simulink model "CarSim_SCANeR_UDP_LKA_THESIS"  (R2019a)
settings: Solver=FixedStepDiscrete  StartTime=0.0  StopTime=inf  FixedStep=0.001  RelTol=1e-3  EnableMultiTasking=on
undefined symbols (not defined in the file or in its folder): DiscIntNeverNeededParam
libraries: simulink x11, xpcutilitieslib x2, xpcrtudplib x2, dspnetwork x1
(part 2 of 2)

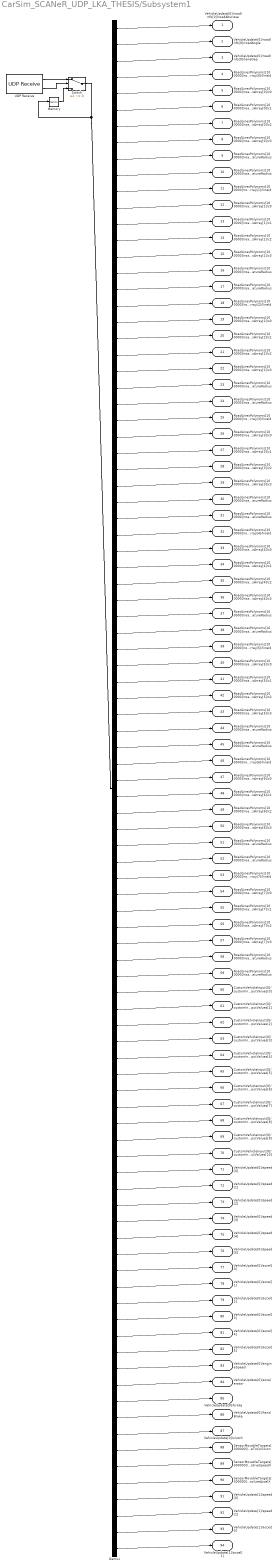
== system CarSim_SCANeR_UDP_LKA_THESIS/Subsystem1 ==
  Demux : Demux  Outputs=94
  Memory : Memory  InheritSampleTime=on
  Switch : Switch  Criteria=u2 ~= 0
  UDP Receive : dspnetwork/UDP Receive  localURL='0.0.0.0'  localPort=8193  remoteURL='0.0.0.0'  remotePort=-1  recvBufferSize=752  dims=94  signalDatatype=double  isComplex=off  isVarSize=off  showBlockingTime=on  blockingTime=0  sampletime=0.01  blockPlatform=HOST
      settings: SourceProductName=Simulink
  VehicleUpdate[0]/roadInfo[0]/roadAbscissa : Outport
  VehicleUpdate[0]/roadInfo[0]/roadAngle : Outport  Port=2
  VehicleUpdate[0]/roadInfo[0]/laneGap : Outport  Port=3
  RoadLinesPolynoms[100000]/roadLinesPolynomsArray[0]/lineId : Outport  Port=4
  RoadLinesPolynoms[100000]/roadLinesPolynomsArray[0]/c0 : Outport  Port=5
  RoadLinesPolynoms[100000]/roadLinesPolynomsArray[0]/c1 : Outport  Port=6
  RoadLinesPolynoms[100000]/roadLinesPolynomsArray[0]/c2 : Outport  Port=7
  RoadLinesPolynoms[100000]/roadLinesPolynomsArray[0]/c3 : Outport  Port=8
  RoadLinesPolynoms[100000]/roadLinesPolynomsArray[0]/curvatureRadius : Outport  Port=9
  RoadLinesPolynoms[100000]/roadLinesPolynomsArray[0]/estimatedCurvatureRadius : Outport  Port=10
  RoadLinesPolynoms[100000]/roadLinesPolynomsArray[1]/lineId : Outport  Port=11
  RoadLinesPolynoms[100000]/roadLinesPolynomsArray[1]/c0 : Outport  Port=12
  RoadLinesPolynoms[100000]/roadLinesPolynomsArray[1]/c1 : Outport  Port=13
  RoadLinesPolynoms[100000]/roadLinesPolynomsArray[1]/c2 : Outport  Port=14
  RoadLinesPolynoms[100000]/roadLinesPolynomsArray[1]/c3 : Outport  Port=15
  RoadLinesPolynoms[100000]/roadLinesPolynomsArray[1]/curvatureRadius : Outport  Port=16
  RoadLinesPolynoms[100000]/roadLinesPolynomsArray[1]/estimatedCurvatureRadius : Outport  Port=17
  RoadLinesPolynoms[100000]/roadLinesPolynomsArray[2]/lineId : Outport  Port=18
  RoadLinesPolynoms[100000]/roadLinesPolynomsArray[2]/c0 : Outport  Port=19
  RoadLinesPolynoms[100000]/roadLinesPolynomsArray[2]/c1 : Outport  Port=20
  RoadLinesPolynoms[100000]/roadLinesPolynomsArray[2]/c2 : Outport  Port=21
  RoadLinesPolynoms[100000]/roadLinesPolynomsArray[2]/c3 : Outport  Port=22
  RoadLinesPolynoms[100000]/roadLinesPolynomsArray[2]/curvatureRadius : Outport  Port=23
  RoadLinesPolynoms[100000]/roadLinesPolynomsArray[2]/estimatedCurvatureRadius : Outport  Port=24
  RoadLinesPolynoms[100000]/roadLinesPolynomsArray[3]/lineId : Outport  Port=25
  RoadLinesPolynoms[100000]/roadLinesPolynomsArray[3]/c0 : Outport  Port=26
  RoadLinesPolynoms[100000]/roadLinesPolynomsArray[3]/c1 : Outport  Port=27
  RoadLinesPolynoms[100000]/roadLinesPolynomsArray[3]/c2 : Outport  Port=28
  RoadLinesPolynoms[100000]/roadLinesPolynomsArray[3]/c3 : Outport  Port=29
  RoadLinesPolynoms[100000]/roadLinesPolynomsArray[3]/curvatureRadius : Outport  Port=30
  RoadLinesPolynoms[100000]/roadLinesPolynomsArray[3]/estimatedCurvatureRadius : Outport  Port=31
  RoadLinesPolynoms[100000]/roadLinesPolynomsArray[4]/lineId : Outport  Port=32
  RoadLinesPolynoms[100000]/roadLinesPolynomsArray[4]/c0 : Outport  Port=33
  RoadLinesPolynoms[100000]/roadLinesPolynomsArray[4]/c1 : Outport  Port=34
  RoadLinesPolynoms[100000]/roadLinesPolynomsArray[4]/c2 : Outport  Port=35
  RoadLinesPolynoms[100000]/roadLinesPolynomsArray[4]/c3 : Outport  Port=36
  RoadLinesPolynoms[100000]/roadLinesPolynomsArray[4]/curvatureRadius : Outport  Port=37
  RoadLinesPolynoms[100000]/roadLinesPolynomsArray[4]/estimatedCurvatureRadius : Outport  Port=38
  RoadLinesPolynoms[100000]/roadLinesPolynomsArray[5]/lineId : Outport  Port=39
  RoadLinesPolynoms[100000]/roadLinesPolynomsArray[5]/c0 : Outport  Port=40
  RoadLinesPolynoms[100000]/roadLinesPolynomsArray[5]/c1 : Outport  Port=41
  RoadLinesPolynoms[100000]/roadLinesPolynomsArray[5]/c2 : Outport  Port=42
  RoadLinesPolynoms[100000]/roadLinesPolynomsArray[5]/c3 : Outport  Port=43
  RoadLinesPolynoms[100000]/roadLinesPolynomsArray[5]/curvatureRadius : Outport  Port=44
  RoadLinesPolynoms[100000]/roadLinesPolynomsArray[5]/estimatedCurvatureRadius : Outport  Port=45
  RoadLinesPolynoms[100000]/roadLinesPolynomsArray[6]/lineId : Outport  Port=46
  RoadLinesPolynoms[100000]/roadLinesPolynomsArray[6]/c0 : Outport  Port=47
  RoadLinesPolynoms[100000]/roadLinesPolynomsArray[6]/c1 : Outport  Port=48
  RoadLinesPolynoms[100000]/roadLinesPolynomsArray[6]/c2 : Outport  Port=49
  RoadLinesPolynoms[100000]/roadLinesPolynomsArray[6]/c3 : Outport  Port=50
  RoadLinesPolynoms[100000]/roadLinesPolynomsArray[6]/curvatureRadius : Outport  Port=51
  RoadLinesPolynoms[100000]/roadLinesPolynomsArray[6]/estimatedCurvatureRadius : Outport  Port=52
  RoadLinesPolynoms[100000]/roadLinesPolynomsArray[7]/lineId : Outport  Port=53
  RoadLinesPolynoms[100000]/roadLinesPolynomsArray[7]/c0 : Outport  Port=54
  RoadLinesPolynoms[100000]/roadLinesPolynomsArray[7]/c1 : Outport  Port=55
  RoadLinesPolynoms[100000]/roadLinesPolynomsArray[7]/c2 : Outport  Port=56
  RoadLinesPolynoms[100000]/roadLinesPolynomsArray[7]/c3 : Outport  Port=57
  RoadLinesPolynoms[100000]/roadLinesPolynomsArray[7]/curvatureRadius : Outport  Port=58
  RoadLinesPolynoms[100000]/roadLinesPolynomsArray[7]/estimatedCurvatureRadius : Outport  Port=59
  CustomVehicleInput[0]/customInputValues[0] : Outport  Port=60
  CustomVehicleInput[0]/customInputValues[1] : Outport  Port=61
  CustomVehicleInput[0]/customInputValues[2] : Outport  Port=62
  CustomVehicleInput[0]/customInputValues[3] : Outport  Port=63
  CustomVehicleInput[0]/customInputValues[4] : Outport  Port=64
  CustomVehicleInput[0]/customInputValues[5] : Outport  Port=65
  CustomVehicleInput[0]/customInputValues[6] : Outport  Port=66
  CustomVehicleInput[0]/customInputValues[7] : Outport  Port=67
  CustomVehicleInput[0]/customInputValues[8] : Outport  Port=68
  CustomVehicleInput[0]/customInputValues[9] : Outport  Port=69
  CustomVehicleInput[0]/customInputValues[10] : Outport  Port=70
  VehicleUpdate[0]/speed[0] : Outport  Port=71
  VehicleUpdate[0]/speed[1] : Outport  Port=72
  VehicleUpdate[0]/speed[2] : Outport  Port=73
  VehicleUpdate[0]/speed[3] : Outport  Port=74
  VehicleUpdate[0]/speed[4] : Outport  Port=75
  VehicleUpdate[0]/speed[5] : Outport  Port=76
  VehicleUpdate[0]/accel[0] : Outport  Port=77
  VehicleUpdate[0]/accel[1] : Outport  Port=78
  VehicleUpdate[0]/accel[2] : Outport  Port=79
  VehicleUpdate[0]/accel[3] : Outport  Port=80
  VehicleUpdate[0]/accel[4] : Outport  Port=81
  VehicleUpdate[0]/accel[5] : Outport  Port=82
  VehicleUpdate[0]/engineSpeed : Outport  Port=83
  VehicleUpdate[0]/accelerator : Outport  Port=84
  VehicleUpdate[0]/brake : Outport  Port=85
  VehicleUpdate[0]/handBrake : Outport  Port=86
  VehicleUpdate[0]/clutch : Outport  Port=87
  SensorMovableTargets[300000]/targetsArray[0]/distanceToCollision : Outport  Port=88
  SensorMovableTargets[300000]/targetsArray[0]/relativeSpeedX : Outport  Port=89
  SensorMovableTargets[300000]/targetsArray[0]/absoluteAccelX : Outport  Port=90
  VehicleUpdate[1]/speed[0] : Outport  Port=91
  VehicleUpdate[1]/speed[1] : Outport  Port=92
  VehicleUpdate[1]/accel[0] : Outport  Port=93
  VehicleUpdate[1]/accel[1] : Outport  Port=94
  wires:
  UDP Receive/1 -> Switch/1
  Demux/1 -> VehicleUpdate[0]/roadInfo[0]/roadAbscissa/1
  Demux/2 -> VehicleUpdate[0]/roadInfo[0]/roadAngle/1
  Demux/3 -> VehicleUpdate[0]/roadInfo[0]/laneGap/1
  Demux/4 -> RoadLinesPolynoms[100000]/roadLinesPolynomsArray[0]/lineId/1
  Demux/5 -> RoadLinesPolynoms[100000]/roadLinesPolynomsArray[0]/c0/1
  Demux/6 -> RoadLinesPolynoms[100000]/roadLinesPolynomsArray[0]/c1/1
  Demux/7 -> RoadLinesPolynoms[100000]/roadLinesPolynomsArray[0]/c2/1
  Demux/8 -> RoadLinesPolynoms[100000]/roadLinesPolynomsArray[0]/c3/1
  Demux/9 -> RoadLinesPolynoms[100000]/roadLinesPolynomsArray[0]/curvatureRadius/1
  Demux/10 -> RoadLinesPolynoms[100000]/roadLinesPolynomsArray[0]/estimatedCurvatureRadius/1
  Demux/11 -> RoadLinesPolynoms[100000]/roadLinesPolynomsArray[1]/lineId/1
  Demux/12 -> RoadLinesPolynoms[100000]/roadLinesPolynomsArray[1]/c0/1
  Demux/13 -> RoadLinesPolynoms[100000]/roadLinesPolynomsArray[1]/c1/1
  Demux/14 -> RoadLinesPolynoms[100000]/roadLinesPolynomsArray[1]/c2/1
  Demux/15 -> RoadLinesPolynoms[100000]/roadLinesPolynomsArray[1]/c3/1
  Demux/16 -> RoadLinesPolynoms[100000]/roadLinesPolynomsArray[1]/curvatureRadius/1
  Demux/17 -> RoadLinesPolynoms[100000]/roadLinesPolynomsArray[1]/estimatedCurvatureRadius/1
  Demux/18 -> RoadLinesPolynoms[100000]/roadLinesPolynomsArray[2]/lineId/1
  Demux/19 -> RoadLinesPolynoms[100000]/roadLinesPolynomsArray[2]/c0/1
  Demux/20 -> RoadLinesPolynoms[100000]/roadLinesPolynomsArray[2]/c1/1
  Demux/21 -> RoadLinesPolynoms[100000]/roadLinesPolynomsArray[2]/c2/1
  Demux/22 -> RoadLinesPolynoms[100000]/roadLinesPolynomsArray[2]/c3/1
  Demux/23 -> RoadLinesPolynoms[100000]/roadLinesPolynomsArray[2]/curvatureRadius/1
  Demux/24 -> RoadLinesPolynoms[100000]/roadLinesPolynomsArray[2]/estimatedCurvatureRadius/1
  Demux/25 -> RoadLinesPolynoms[100000]/roadLinesPolynomsArray[3]/lineId/1
  Demux/26 -> RoadLinesPolynoms[100000]/roadLinesPolynomsArray[3]/c0/1
  Demux/27 -> RoadLinesPolynoms[100000]/roadLinesPolynomsArray[3]/c1/1
  Demux/28 -> RoadLinesPolynoms[100000]/roadLinesPolynomsArray[3]/c2/1
  Demux/29 -> RoadLinesPolynoms[100000]/roadLinesPolynomsArray[3]/c3/1
  Demux/30 -> RoadLinesPolynoms[100000]/roadLinesPolynomsArray[3]/curvatureRadius/1
  Demux/31 -> RoadLinesPolynoms[100000]/roadLinesPolynomsArray[3]/estimatedCurvatureRadius/1
  Demux/32 -> RoadLinesPolynoms[100000]/roadLinesPolynomsArray[4]/lineId/1
  Demux/33 -> RoadLinesPolynoms[100000]/roadLinesPolynomsArray[4]/c0/1
  Demux/34 -> RoadLinesPolynoms[100000]/roadLinesPolynomsArray[4]/c1/1
  Demux/35 -> RoadLinesPolynoms[100000]/roadLinesPolynomsArray[4]/c2/1
  Demux/36 -> RoadLinesPolynoms[100000]/roadLinesPolynomsArray[4]/c3/1
  Demux/37 -> RoadLinesPolynoms[100000]/roadLinesPolynomsArray[4]/curvatureRadius/1
  Demux/38 -> RoadLinesPolynoms[100000]/roadLinesPolynomsArray[4]/estimatedCurvatureRadius/1
  Demux/39 -> RoadLinesPolynoms[100000]/roadLinesPolynomsArray[5]/lineId/1
  Demux/40 -> RoadLinesPolynoms[100000]/roadLinesPolynomsArray[5]/c0/1
  Demux/41 -> RoadLinesPolynoms[100000]/roadLinesPolynomsArray[5]/c1/1
  Demux/42 -> RoadLinesPolynoms[100000]/roadLinesPolynomsArray[5]/c2/1
  Demux/43 -> RoadLinesPolynoms[100000]/roadLinesPolynomsArray[5]/c3/1
  Demux/44 -> RoadLinesPolynoms[100000]/roadLinesPolynomsArray[5]/curvatureRadius/1
  Demux/45 -> RoadLinesPolynoms[100000]/roadLinesPolynomsArray[5]/estimatedCurvatureRadius/1
  Demux/46 -> RoadLinesPolynoms[100000]/roadLinesPolynomsArray[6]/lineId/1
  Demux/47 -> RoadLinesPolynoms[100000]/roadLinesPolynomsArray[6]/c0/1
  Demux/48 -> RoadLinesPolynoms[100000]/roadLinesPolynomsArray[6]/c1/1
  Demux/49 -> RoadLinesPolynoms[100000]/roadLinesPolynomsArray[6]/c2/1
  Demux/50 -> RoadLinesPolynoms[100000]/roadLinesPolynomsArray[6]/c3/1
  Demux/51 -> RoadLinesPolynoms[100000]/roadLinesPolynomsArray[6]/curvatureRadius/1
  Demux/52 -> RoadLinesPolynoms[100000]/roadLinesPolynomsArray[6]/estimatedCurvatureRadius/1
  Demux/53 -> RoadLinesPolynoms[100000]/roadLinesPolynomsArray[7]/lineId/1
  Demux/54 -> RoadLinesPolynoms[100000]/roadLinesPolynomsArray[7]/c0/1
  Demux/55 -> RoadLinesPolynoms[100000]/roadLinesPolynomsArray[7]/c1/1
  Demux/56 -> RoadLinesPolynoms[100000]/roadLinesPolynomsArray[7]/c2/1
  Demux/57 -> RoadLinesPolynoms[100000]/roadLinesPolynomsArray[7]/c3/1
  Demux/58 -> RoadLinesPolynoms[100000]/roadLinesPolynomsArray[7]/curvatureRadius/1
  Demux/59 -> RoadLinesPolynoms[100000]/roadLinesPolynomsArray[7]/estimatedCurvatureRadius/1
  Demux/60 -> CustomVehicleInput[0]/customInputValues[0]/1
  Demux/61 -> CustomVehicleInput[0]/customInputValues[1]/1
  Demux/62 -> CustomVehicleInput[0]/customInputValues[2]/1
  Demux/63 -> CustomVehicleInput[0]/customInputValues[3]/1
  Demux/64 -> CustomVehicleInput[0]/customInputValues[4]/1
  Demux/65 -> CustomVehicleInput[0]/customInputValues[5]/1
  Demux/66 -> CustomVehicleInput[0]/customInputValues[6]/1
  Demux/67 -> CustomVehicleInput[0]/customInputValues[7]/1
  Demux/68 -> CustomVehicleInput[0]/customInputValues[8]/1
  Demux/69 -> CustomVehicleInput[0]/customInputValues[9]/1
  Demux/70 -> CustomVehicleInput[0]/customInputValues[10]/1
  Demux/71 -> VehicleUpdate[0]/speed[0]/1
  Demux/72 -> VehicleUpdate[0]/speed[1]/1
  Demux/73 -> VehicleUpdate[0]/speed[2]/1
  Demux/74 -> VehicleUpdate[0]/speed[3]/1
  Demux/75 -> VehicleUpdate[0]/speed[4]/1
  Demux/76 -> VehicleUpdate[0]/speed[5]/1
  Demux/77 -> VehicleUpdate[0]/accel[0]/1
  Demux/78 -> VehicleUpdate[0]/accel[1]/1
  Demux/79 -> VehicleUpdate[0]/accel[2]/1
  Demux/80 -> VehicleUpdate[0]/accel[3]/1
  Demux/81 -> VehicleUpdate[0]/accel[4]/1
  Demux/82 -> VehicleUpdate[0]/accel[5]/1
  Demux/83 -> VehicleUpdate[0]/engineSpeed/1
  Demux/84 -> VehicleUpdate[0]/accelerator/1
  Demux/85 -> VehicleUpdate[0]/brake/1
  Demux/86 -> VehicleUpdate[0]/handBrake/1
  Demux/87 -> VehicleUpdate[0]/clutch/1
  Demux/88 -> SensorMovableTargets[300000]/targetsArray[0]/distanceToCollision/1
  Demux/89 -> SensorMovableTargets[300000]/targetsArray[0]/relativeSpeedX/1
  Demux/90 -> SensorMovableTargets[300000]/targetsArray[0]/absoluteAccelX/1
  Demux/91 -> VehicleUpdate[1]/speed[0]/1
  Demux/92 -> VehicleUpdate[1]/speed[1]/1
  Demux/93 -> VehicleUpdate[1]/accel[0]/1
  Demux/94 -> VehicleUpdate[1]/accel[1]/1
  UDP Receive/2 -> Switch/2
  Switch/1 -> Memory/1, Demux/1
  Memory/1 -> Switch/3

== system CarSim_SCANeR_UDP_LKA_THESIS/LaneKeep/Subsystem ==
  In1 : Inport
  Enable : EnablePort
  S-Function : S-Function  FunctionName=casadi_fun_lka  Parameters='lka.casadi', 'lka'  SFunctionDeploymentMode=off  EnableBusSupport=off
  Steer : Outport
  wires:
  In1/1 -> S-Function/1
  S-Function/1 -> Steer/1  "Steer"

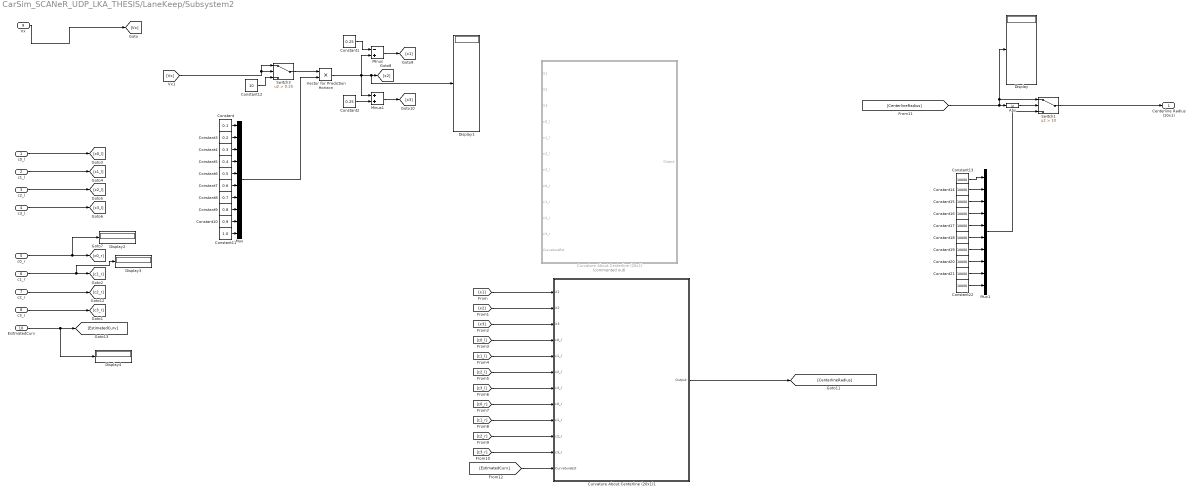
== system CarSim_SCANeR_UDP_LKA_THESIS/LaneKeep/Subsystem2 ==
  c0_l : Inport
  c1_l : Inport  Port=2
  c2_l : Inport  Port=3
  c3_l : Inport  Port=4
  c0_r : Inport  Port=5
  c1_r : Inport  Port=6
  c2_r : Inport  Port=7
  c3_r : Inport  Port=8
  Vx : Inport  Port=9
  EsitmatedCurv : Inport  Port=10
  Abs : Abs
  Constant : Constant  Value=0.1
  Constant1 : Constant  Value=0.25
  Constant10 : Constant  Value=0.9
  Constant11 : Constant  Value=1.0
  Constant12 : Constant  Value=10
  Constant{13..22} (10 alike) : Constant  Value=10000
  Constant2 : Constant  Value=0.25
  Constant3 : Constant  Value=0.2
  Constant4 : Constant  Value=0.3
  Constant5 : Constant  Value=0.4
  Constant6 : Constant  Value=0.5
  Constant7 : Constant  Value=0.6
  Constant8 : Constant  Value=0.7
  Constant9 : Constant  Value=0.8
  Curvature About Centerline (20x1) : Subsystem  Commented=on  TreatAsAtomicUnit=on
  Curvature About Centerline (20x1)1 : Subsystem
      mask help: Simulink:masks:GenSFuncDesc_MD
      mask Help: eval('feval(''rtwprivate'',''rtwhelpview'',''rtw_sfcn_block'')');
  Display{,1..4} (5 alike) : Display
  Minus : Sum  Inputs=-+
  Minus1 : Sum
  Mux : Mux  Inputs=10
  Mux1 : Mux  Inputs=10
  Switch1 : Switch  Criteria=u2 > Threshold  Threshold=10
  Switch3 : Switch  Criteria=u2 > Threshold  Threshold=0.25
  Vector for Prediction Horizon : Product  Inputs=**
  Centerline Radius (10x1) : Outport  VectorParamsAs1DForOutWhenUnconnected=on
  wires:
  Mux1/1 -> Switch1/3
  Constant13/1 -> Mux1/1
  Constant14/1 -> Mux1/2
  Constant15/1 -> Mux1/3
  Constant16/1 -> Mux1/4
  Constant17/1 -> Mux1/5
  Constant18/1 -> Mux1/6
  Constant19/1 -> Mux1/7
  Constant20/1 -> Mux1/8
  Constant21/1 -> Mux1/9
  Constant22/1 -> Mux1/10
  Switch1/1 -> Centerline Radius (10x1)/1
  [CenterlineRadius] -> Abs/1, Display/1, Switch1/1
  Constant11/1 -> Mux/10
  Constant10/1 -> Mux/9
  Constant9/1 -> Mux/8
  Constant8/1 -> Mux/7
  Constant7/1 -> Mux/6
  Constant6/1 -> Mux/5
  Constant5/1 -> Mux/4
  Constant4/1 -> Mux/3
  Constant3/1 -> Mux/2
  Constant/1 -> Mux/1
  Constant12/1 -> Switch3/3
  Mux/1 -> Vector for Prediction Horizon/2
  Switch3/1 -> Vector for Prediction Horizon/1
  c3_l/1 -> [c3_l]
  c0_r/1 -> Display2/1, [c0_r]
  c0_l/1 -> [c0_l]
  c1_l/1 -> [c1_l]
  c2_l/1 -> [c2_l]
  c1_r/1 -> Display3/1, [c1_r]
  c2_r/1 -> [c2_r]
  c3_r/1 -> [c3_r]
  Minus/1 -> [x1]
  Constant1/1 -> Minus/1
  Constant2/1 -> Minus1/2
  Minus1/1 -> [x3]
  Vector for Prediction Horizon/1 -> Minus1/1, Display1/1, [x2], Minus/2
  [Vx] -> Switch3/2, Switch3/1
  Vx/1 -> [Vx]
  EsitmatedCurv/1 -> Display4/1, [EstimatedCurv]
  Abs/1 -> Switch1/2
  Curvature About Centerline (20x1)1/1(Output) -> [CenterlineRadius]
  [x1] -> Curvature About Centerline (20x1)1/1(X1)
  [x2] -> Curvature About Centerline (20x1)1/2(X2)
  [x3] -> Curvature About Centerline (20x1)1/3(X3)
  [c0_l] -> Curvature About Centerline (20x1)1/4(c0_l)
  [c1_l] -> Curvature About Centerline (20x1)1/5(c1_l)
  [c2_l] -> Curvature About Centerline (20x1)1/6(c2_l)
  [c3_l] -> Curvature About Centerline (20x1)1/7(c3_l)
  [c0_r] -> Curvature About Centerline (20x1)1/8(c0_r)
  [c1_r] -> Curvature About Centerline (20x1)1/9(c1_r)
  [c2_r] -> Curvature About Centerline (20x1)1/10(c2_r)
  [c3_r] -> Curvature About Centerline (20x1)1/11(c3_r)
  [EstimatedCurv] -> Curvature About Centerline (20x1)1/12(" CurvatureEst")

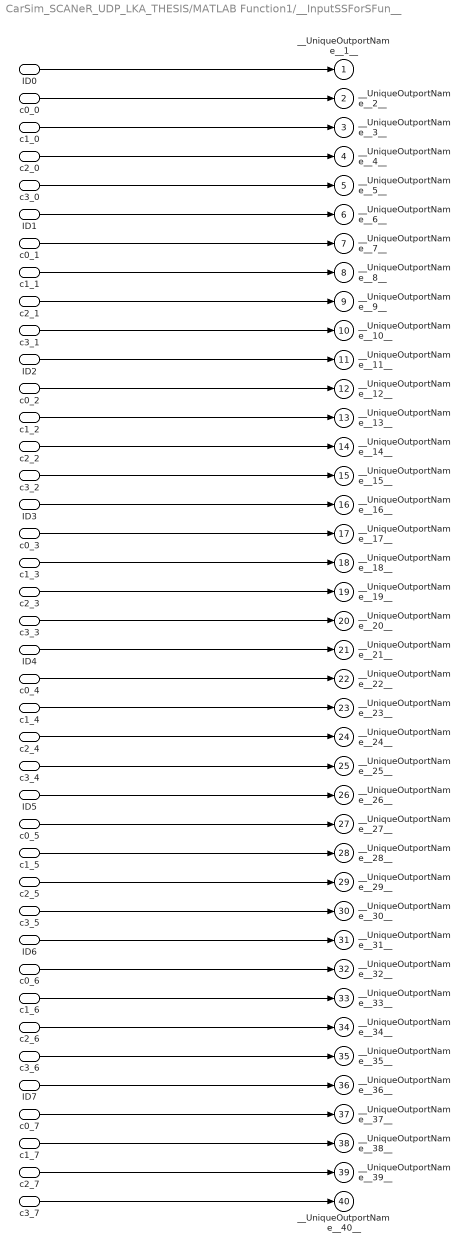
== system CarSim_SCANeR_UDP_LKA_THESIS/MATLAB Function1/__InputSSForSFun__ ==
  ID0 : Inport
  c0_0 : Inport  Port=2
  c1_0 : Inport  Port=3
  c2_0 : Inport  Port=4
  c3_0 : Inport  Port=5
  ID1 : Inport  Port=6
  c0_1 : Inport  Port=7
  c1_1 : Inport  Port=8
  c2_1 : Inport  Port=9
  c3_1 : Inport  Port=10
  ID2 : Inport  Port=11
  c0_2 : Inport  Port=12
  c1_2 : Inport  Port=13
  c2_2 : Inport  Port=14
  c3_2 : Inport  Port=15
  ID3 : Inport  Port=16
  c0_3 : Inport  Port=17
  c1_3 : Inport  Port=18
  c2_3 : Inport  Port=19
  c3_3 : Inport  Port=20
  ID4 : Inport  Port=21
  c0_4 : Inport  Port=22
  c1_4 : Inport  Port=23
  c2_4 : Inport  Port=24
  c3_4 : Inport  Port=25
  ID5 : Inport  Port=26
  c0_5 : Inport  Port=27
  c1_5 : Inport  Port=28
  c2_5 : Inport  Port=29
  c3_5 : Inport  Port=30
  ID6 : Inport  Port=31
  c0_6 : Inport  Port=32
  c1_6 : Inport  Port=33
  c2_6 : Inport  Port=34
  c3_6 : Inport  Port=35
  ID7 : Inport  Port=36
  c0_7 : Inport  Port=37
  c1_7 : Inport  Port=38
  c2_7 : Inport  Port=39
  c3_7 : Inport  Port=40
  __UniqueOutportName__1__ : Outport
  __UniqueOutportName__2__ : Outport  Port=2
  __UniqueOutportName__3__ : Outport  Port=3
  __UniqueOutportName__4__ : Outport  Port=4
  __UniqueOutportName__5__ : Outport  Port=5
  __UniqueOutportName__6__ : Outport  Port=6
  __UniqueOutportName__7__ : Outport  Port=7
  __UniqueOutportName__8__ : Outport  Port=8
  __UniqueOutportName__9__ : Outport  Port=9
  __UniqueOutportName__10__ : Outport  Port=10
  __UniqueOutportName__11__ : Outport  Port=11
  __UniqueOutportName__12__ : Outport  Port=12
  __UniqueOutportName__13__ : Outport  Port=13
  __UniqueOutportName__14__ : Outport  Port=14
  __UniqueOutportName__15__ : Outport  Port=15
  __UniqueOutportName__16__ : Outport  Port=16
  __UniqueOutportName__17__ : Outport  Port=17
  __UniqueOutportName__18__ : Outport  Port=18
  __UniqueOutportName__19__ : Outport  Port=19
  __UniqueOutportName__20__ : Outport  Port=20
  __UniqueOutportName__21__ : Outport  Port=21
  __UniqueOutportName__22__ : Outport  Port=22
  __UniqueOutportName__23__ : Outport  Port=23
  __UniqueOutportName__24__ : Outport  Port=24
  __UniqueOutportName__25__ : Outport  Port=25
  __UniqueOutportName__26__ : Outport  Port=26
  __UniqueOutportName__27__ : Outport  Port=27
  __UniqueOutportName__28__ : Outport  Port=28
  __UniqueOutportName__29__ : Outport  Port=29
  __UniqueOutportName__30__ : Outport  Port=30
  __UniqueOutportName__31__ : Outport  Port=31
  __UniqueOutportName__32__ : Outport  Port=32
  __UniqueOutportName__33__ : Outport  Port=33
  __UniqueOutportName__34__ : Outport  Port=34
  __UniqueOutportName__35__ : Outport  Port=35
  __UniqueOutportName__36__ : Outport  Port=36
  __UniqueOutportName__37__ : Outport  Port=37
  __UniqueOutportName__38__ : Outport  Port=38
  __UniqueOutportName__39__ : Outport  Port=39
  __UniqueOutportName__40__ : Outport  Port=40
  wires:
  ID0/1 -> __UniqueOutportName__1__/1
  c0_0/1 -> __UniqueOutportName__2__/1
  c1_0/1 -> __UniqueOutportName__3__/1
  c2_0/1 -> __UniqueOutportName__4__/1
  c3_0/1 -> __UniqueOutportName__5__/1
  ID1/1 -> __UniqueOutportName__6__/1
  c0_1/1 -> __UniqueOutportName__7__/1
  c1_1/1 -> __UniqueOutportName__8__/1
  c2_1/1 -> __UniqueOutportName__9__/1
  c3_1/1 -> __UniqueOutportName__10__/1
  ID2/1 -> __UniqueOutportName__11__/1
  c0_2/1 -> __UniqueOutportName__12__/1
  c1_2/1 -> __UniqueOutportName__13__/1
  c2_2/1 -> __UniqueOutportName__14__/1
  c3_2/1 -> __UniqueOutportName__15__/1
  ID3/1 -> __UniqueOutportName__16__/1
  c0_3/1 -> __UniqueOutportName__17__/1
  c1_3/1 -> __UniqueOutportName__18__/1
  c2_3/1 -> __UniqueOutportName__19__/1
  c3_3/1 -> __UniqueOutportName__20__/1
  ID4/1 -> __UniqueOutportName__21__/1
  c0_4/1 -> __UniqueOutportName__22__/1
  c1_4/1 -> __UniqueOutportName__23__/1
  c2_4/1 -> __UniqueOutportName__24__/1
  c3_4/1 -> __UniqueOutportName__25__/1
  ID5/1 -> __UniqueOutportName__26__/1
  c0_5/1 -> __UniqueOutportName__27__/1
  c1_5/1 -> __UniqueOutportName__28__/1
  c2_5/1 -> __UniqueOutportName__29__/1
  c3_5/1 -> __UniqueOutportName__30__/1
  ID6/1 -> __UniqueOutportName__31__/1
  c0_6/1 -> __UniqueOutportName__32__/1
  c1_6/1 -> __UniqueOutportName__33__/1
  c2_6/1 -> __UniqueOutportName__34__/1
  c3_6/1 -> __UniqueOutportName__35__/1
  ID7/1 -> __UniqueOutportName__36__/1
  c0_7/1 -> __UniqueOutportName__37__/1
  c1_7/1 -> __UniqueOutportName__38__/1
  c2_7/1 -> __UniqueOutportName__39__/1
  c3_7/1 -> __UniqueOutportName__40__/1

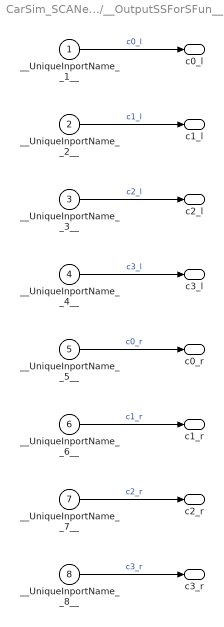
== system CarSim_SCANeR_UDP_LKA_THESIS/MATLAB Function1/__OutputSSForSFun__ ==
  __UniqueInportName__1__ : Inport
  __UniqueInportName__2__ : Inport  Port=2
  __UniqueInportName__3__ : Inport  Port=3
  __UniqueInportName__4__ : Inport  Port=4
  __UniqueInportName__5__ : Inport  Port=5
  __UniqueInportName__6__ : Inport  Port=6
  __UniqueInportName__7__ : Inport  Port=7
  __UniqueInportName__8__ : Inport  Port=8
  c0_l : Outport
  c1_l : Outport  Port=2
  c2_l : Outport  Port=3
  c3_l : Outport  Port=4
  c0_r : Outport  Port=5
  c1_r : Outport  Port=6
  c2_r : Outport  Port=7
  c3_r : Outport  Port=8
  wires:
  __UniqueInportName__1__/1 -> c0_l/1  "c0_l"
  __UniqueInportName__2__/1 -> c1_l/1  "c1_l"
  __UniqueInportName__3__/1 -> c2_l/1  "c2_l"
  __UniqueInportName__4__/1 -> c3_l/1  "c3_l"
  __UniqueInportName__5__/1 -> c0_r/1  "c0_r"
  __UniqueInportName__6__/1 -> c1_r/1  "c1_r"
  __UniqueInportName__7__/1 -> c2_r/1  "c2_r"
  __UniqueInportName__8__/1 -> c3_r/1  "c3_r"

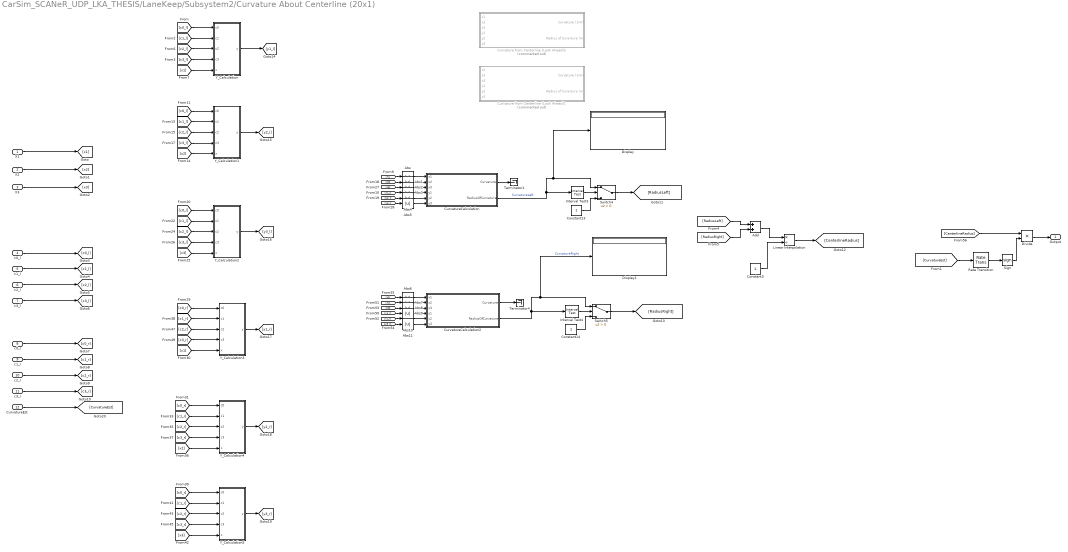
== system CarSim_SCANeR_UDP_LKA_THESIS/LaneKeep/Subsystem2/Curvature About Centerline (20x1) ==
  X1 : Inport
  X2 : Inport  Port=2
  X3 : Inport  Port=3
  c0_l : Inport  Port=4
  c1_l : Inport  Port=5
  c2_l : Inport  Port=6
  c3_l : Inport  Port=7
  c0_r : Inport  Port=8
  c1_r : Inport  Port=9
  c2_r : Inport  Port=10
  c3_r : Inport  Port=11
  " CurvatureEst" : Inport  Port=12
  Abs{,1..11} (12 alike) : Abs
  Add : Sum
  Constant13 : Constant
  Constant14 : Constant
  Constant5 : Constant  Value=2
  Curvature from Centerline (Look Ahead)1 : Subsystem  Commented=on
  Curvature from Centerline (Look Ahead)2 : Subsystem  Commented=on
  CurvatureCalculation : MATLAB Function  TreatAsAtomicUnit=on
  CurvatureCalculation2 : MATLAB Function  TreatAsAtomicUnit=on
  Display : Display
  Display1 : Display
  Divide : Product  Inputs=**
  Interval Test3 : simulink/Logic and Bit Operations/Interval Test  IntervalClosedRight=on  uplimit=1000000000  IntervalClosedLeft=on  lowlimit=-100000000  OutDataTypeStr=boolean
  Interval Test4 : simulink/Logic and Bit Operations/Interval Test  IntervalClosedRight=on  uplimit=100000000  IntervalClosedLeft=on  lowlimit=-100000000  OutDataTypeStr=boolean
  Linear Interpolation : Product  Inputs=*/
  Rate Transition : RateTransition
  Sign : Signum
  Switch4 : Switch  Criteria=u2 > Threshold
  Switch5 : Switch  Criteria=u2 > Threshold
  Terminator1 : Terminator
  Terminator4 : Terminator
  Y_Calculation : MATLAB Function  TreatAsAtomicUnit=on
  Y_Calculation1 : MATLAB Function  TreatAsAtomicUnit=on
  Y_Calculation2 : MATLAB Function  TreatAsAtomicUnit=on
  Y_Calculation3 : MATLAB Function  TreatAsAtomicUnit=on
  Y_Calculation4 : MATLAB Function  TreatAsAtomicUnit=on
  Y_Calculation5 : MATLAB Function  TreatAsAtomicUnit=on
  Output : Outport
  wires:
  Abs11/1 -> CurvatureCalculation2/6(y3)
  Abs10/1 -> CurvatureCalculation2/5(y2)
  Abs9/1 -> CurvatureCalculation2/4(y1)
  Abs8/1 -> CurvatureCalculation2/3(x3)
  Abs7/1 -> CurvatureCalculation2/2(x2)
  Abs6/1 -> CurvatureCalculation2/1(x1)
  Abs5/1 -> CurvatureCalculation/6(y3)
  Abs4/1 -> CurvatureCalculation/5(y2)
  Abs3/1 -> CurvatureCalculation/4(y1)
  Abs2/1 -> CurvatureCalculation/3(x3)
  Abs1/1 -> CurvatureCalculation/2(x2)
  Abs/1 -> CurvatureCalculation/1(x1)
  CurvatureCalculation2/1(Curvature) -> Terminator4/1
  CurvatureCalculation/1(Curvature) -> Terminator1/1
  [x3] -> Y_Calculation5/5(x)
  [c3_r] -> Y_Calculation5/4(c3)
  [c2_r] -> Y_Calculation5/3(c2)
  [c1_r] -> Y_Calculation5/2(c1)
  [c0_r] -> Y_Calculation5/1(c0)
  [x2] -> Y_Calculation4/5(x)
  [c3_r] -> Y_Calculation4/4(c3)
  [c2_r] -> Y_Calculation4/3(c2)
  [c1_r] -> Y_Calculation4/2(c1)
  [c0_r] -> Y_Calculation4/1(c0)
  [x1] -> Y_Calculation3/5(x)
  [c3_r] -> Y_Calculation3/4(c3)
  [c2_r] -> Y_Calculation3/3(c2)
  [c1_r] -> Y_Calculation3/2(c1)
  [c0_r] -> Y_Calculation3/1(c0)
  Y_Calculation5/1(y) -> [y3_r]
  Y_Calculation4/1(y) -> [y2_r]
  Y_Calculation3/1(y) -> [y1_r]
  Y_Calculation2/1(y) -> [y3_l]
  [x3] -> Y_Calculation2/5(x)
  [c3_l] -> Y_Calculation2/4(c3)
  [c2_l] -> Y_Calculation2/3(c2)
  [c1_l] -> Y_Calculation2/2(c1)
  [c0_l] -> Y_Calculation2/1(c0)
  Y_Calculation1/1(y) -> [y2_l]
  [x2] -> Y_Calculation1/5(x)
  [c3_l] -> Y_Calculation1/4(c3)
  [c2_l] -> Y_Calculation1/3(c2)
  [c1_l] -> Y_Calculation1/2(c1)
  [c0_l] -> Y_Calculation1/1(c0)
  [x1] -> Y_Calculation/5(x)
  [c3_l] -> Y_Calculation/4(c3)
  [c2_l] -> Y_Calculation/3(c2)
  [c1_l] -> Y_Calculation/2(c1)
  [c0_l] -> Y_Calculation/1(c0)
  Y_Calculation/1(y) -> [y1_l]
  [y3_r] -> Abs11/1
  [y2_r] -> Abs10/1
  [y1_r] -> Abs9/1
  [x3] -> Abs8/1
  [x2] -> Abs7/1
  [x1] -> Abs6/1
  [y3_l] -> Abs5/1
  [y2_l] -> Abs4/1
  [y1_l] -> Abs3/1
  [x3] -> Abs2/1
  [x2] -> Abs1/1
  [x1] -> Abs/1
  Divide/1 -> Output/1
  c0_r/1 -> [c0_r]
  c1_r/1 -> [c1_r]
  c2_r/1 -> [c2_r]
  c3_r/1 -> [c3_r]
  c3_l/1 -> [c3_l]
  c2_l/1 -> [c2_l]
  c1_l/1 -> [c1_l]
  c0_l/1 -> [c0_l]
  X3/1 -> [x3]
  X2/1 -> [x2]
  X1/1 -> [x1]
  Add/1 -> Linear Interpolation/1
  [RadiusLeft] -> Add/1
  Constant5/1 -> Linear Interpolation/2
  [RadiusRight] -> Add/2
  Constant13/1 -> Switch4/3
  Switch5/1 -> [RadiusRight]
  Interval Test4/1 -> Switch5/2
  Constant14/1 -> Switch5/3
  Switch4/1 -> [RadiusLeft]
  Linear Interpolation/1 -> [CenterlineRadius]
  CurvatureCalculation/2(RadiusOfCurvature) -> Interval Test3/1, Switch4/1, Display/1  "CurvatureLeft"
  Interval Test3/1 -> Switch4/2
  CurvatureCalculation2/2(RadiusOfCurvature) -> Switch5/1, Display1/1, Interval Test4/1  "CurvatureRight"
  " CurvatureEst"/1 -> [CurvatureEst]
  [CurvatureEst] -> Rate Transition/1
  [CenterlineRadius] -> Divide/1
  Rate Transition/1 -> Sign/1
  Sign/1 -> Divide/2

== system CarSim_SCANeR_UDP_LKA_THESIS/LaneKeep/Subsystem2/Curvature About Centerline (20x1)1 ==
  X1 : Inport
  X2 : Inport  Port=2
  X3 : Inport  Port=3
  c0_l : Inport  Port=4
  c1_l : Inport  Port=5
  c2_l : Inport  Port=6
  c3_l : Inport  Port=7
  c0_r : Inport  Port=8
  c1_r : Inport  Port=9
  c2_r : Inport  Port=10
  c3_r : Inport  Port=11
  " CurvatureEst" : Inport  Port=12
  Curvature About Centerline (20x1)_sfcn : S-Function  FunctionName=Curvature_sf  SFunctionModules=""  SFunctionDeploymentMode=off  EnableBusSupport=off  mask{rtw_sf_name=Curvature_sf, showVar=off}
      mask prompts: rtw_sf_name "Simulink:masks:GenSFuncName_MP"; showVar "Simulink:masks:GenSFuncShowModuleList_MP"
      mask help: Simulink:masks:GenSFuncDesc_MD
      mask init: same as CarSim_SCANeR_UDP_LKA_THESIS/MATLAB Function1/MATLAB Function_sfcn
      settings: CopyFcn=|
      | if ~strcmp(get_param(gcb,'Linkstatus'),'none') && ...
      | ~strcmp(get_param(gcb,'Linkstatus'),'implicit')
      |   set_param(gcb,'LinkStatus','none');
      | end
      mask Help: eval('feval(''rtwprivate'',''rtwhelpview'',''rtw_sfcn_block'')');
      mask Display:
      | port_label('input',1,'X1');
      | port_label('input',2,'X2');
      | port_label('input',3,'X3');
      | port_label('input',4,'c0_l');
      | port_label('input',5,'c1_l');
      | port_label('input',6,'c2_l');
      | port_label('input',7,'c3_l');
      | port_label('input',8,'c0_r');
      | port_label('input',9,'c1_r');
      | port_label('input',10,'c2_r');
      | port_label('input',11,'c3_r');
      | port_label('input',12,' CurvatureEst');
      | port_label('output',1,'Output');
  __InputSSForSFun__ : Subsystem
  __OutputSSForSFun__ : Subsystem
  Output : Outport
  wires:
  __OutputSSForSFun__/1(Output) -> Output/1
  Curvature About Centerline (20x1)_sfcn/1 -> __OutputSSForSFun__/1(__UniqueInportName__1__)
  __InputSSForSFun__/12(__UniqueOutportName__12__) -> Curvature About Centerline (20x1)_sfcn/12
  __InputSSForSFun__/11(__UniqueOutportName__11__) -> Curvature About Centerline (20x1)_sfcn/11
  __InputSSForSFun__/10(__UniqueOutportName__10__) -> Curvature About Centerline (20x1)_sfcn/10
  __InputSSForSFun__/9(__UniqueOutportName__9__) -> Curvature About Centerline (20x1)_sfcn/9
  __InputSSForSFun__/8(__UniqueOutportName__8__) -> Curvature About Centerline (20x1)_sfcn/8
  __InputSSForSFun__/7(__UniqueOutportName__7__) -> Curvature About Centerline (20x1)_sfcn/7
  __InputSSForSFun__/6(__UniqueOutportName__6__) -> Curvature About Centerline (20x1)_sfcn/6
  __InputSSForSFun__/5(__UniqueOutportName__5__) -> Curvature About Centerline (20x1)_sfcn/5
  __InputSSForSFun__/4(__UniqueOutportName__4__) -> Curvature About Centerline (20x1)_sfcn/4
  __InputSSForSFun__/3(__UniqueOutportName__3__) -> Curvature About Centerline (20x1)_sfcn/3
  __InputSSForSFun__/2(__UniqueOutportName__2__) -> Curvature About Centerline (20x1)_sfcn/2
  __InputSSForSFun__/1(__UniqueOutportName__1__) -> Curvature About Centerline (20x1)_sfcn/1
  " CurvatureEst"/1 -> __InputSSForSFun__/12(" CurvatureEst")
  c3_r/1 -> __InputSSForSFun__/11(c3_r)
  c2_r/1 -> __InputSSForSFun__/10(c2_r)
  c1_r/1 -> __InputSSForSFun__/9(c1_r)
  c0_r/1 -> __InputSSForSFun__/8(c0_r)
  c3_l/1 -> __InputSSForSFun__/7(c3_l)
  c2_l/1 -> __InputSSForSFun__/6(c2_l)
  c1_l/1 -> __InputSSForSFun__/5(c1_l)
  c0_l/1 -> __InputSSForSFun__/4(c0_l)
  X3/1 -> __InputSSForSFun__/3(X3)
  X2/1 -> __InputSSForSFun__/2(X2)
  X1/1 -> __InputSSForSFun__/1(X1)

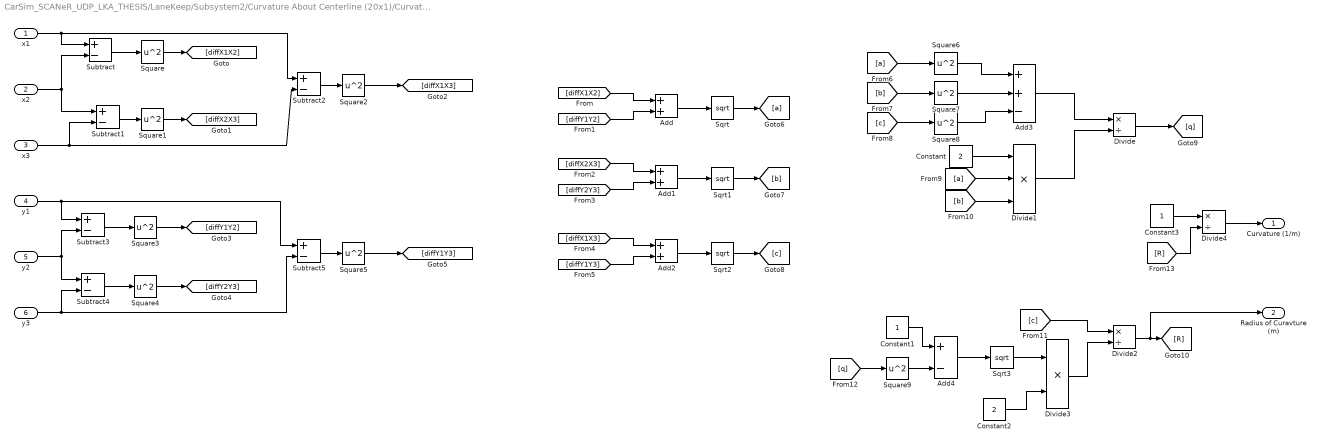
== system CarSim_SCANeR_UDP_LKA_THESIS/LaneKeep/Subsystem2/Curvature About Centerline (20x1)/Curvature from Centerline (Look Ahead)1 ==
  x1 : Inport
  x2 : Inport  Port=2
  x3 : Inport  Port=3
  y1 : Inport  Port=4
  y2 : Inport  Port=5
  y3 : Inport  Port=6
  Add : Sum
  Add1 : Sum
  Add2 : Sum
  Add3 : Sum  Inputs=++-
  Add4 : Sum  Inputs=+-
  Constant : Constant  Value=2
  Constant1 : Constant
  Constant2 : Constant  Value=2
  Constant3 : Constant
  Divide : Product  Inputs=*/
  Divide1 : Product  Inputs=***
  Divide2 : Product  Inputs=*/
  Divide3 : Product  Inputs=**
  Divide4 : Product  Inputs=*/
  Sqrt{,1..3} (4 alike) : Sqrt  SaturateOnIntegerOverflow=on
  Square{,1..9} (10 alike) : Math  Operator=square  SaturateOnIntegerOverflow=on
  Subtract{,1..5} (6 alike) : Sum  Inputs=+-
  "Curvature (1/m) " : Outport  VectorParamsAs1DForOutWhenUnconnected=on
  Radius of Curavture (m) : Outport  Port=2  VectorParamsAs1DForOutWhenUnconnected=on
  wires:
  Divide4/1 -> "Curvature (1/m) "/1
  [R] -> Divide4/2
  Constant3/1 -> Divide4/1
  Divide2/1 -> Radius of Curavture (m)/1, [R]
  Divide3/1 -> Divide2/2
  Constant2/1 -> Divide3/2
  Sqrt3/1 -> Divide3/1
  Add4/1 -> Sqrt3/1
  Constant1/1 -> Add4/1
  Square9/1 -> Add4/2
  [q] -> Square9/1
  [c] -> Divide2/1
  Divide/1 -> [q]
  Divide1/1 -> Divide/2
  [b] -> Divide1/3
  [a] -> Divide1/2
  Constant/1 -> Divide1/1
  Add3/1 -> Divide/1
  Square8/1 -> Add3/3
  [c] -> Square8/1
  Square7/1 -> Add3/2
  [b] -> Square7/1
  Square6/1 -> Add3/1
  [a] -> Square6/1
  Sqrt2/1 -> [c]
  Add2/1 -> Sqrt2/1
  [diffY1Y3] -> Add2/2
  [diffX1X3] -> Add2/1
  [diffX2X3] -> Add1/1
  [diffY2Y3] -> Add1/2
  Add1/1 -> Sqrt1/1
  Sqrt1/1 -> [b]
  Sqrt/1 -> [a]
  Add/1 -> Sqrt/1
  [diffY1Y2] -> Add/2
  [diffX1X2] -> Add/1
  Square5/1 -> [diffY1Y3]
  Square4/1 -> [diffY2Y3]
  Square3/1 -> [diffY1Y2]
  Subtract5/1 -> Square5/1
  y3/1 -> Subtract4/2, Subtract5/2
  Subtract4/1 -> Square4/1
  y2/1 -> Subtract3/2, Subtract4/1
  y1/1 -> Subtract3/1, Subtract5/1
  Subtract3/1 -> Square3/1
  Square2/1 -> [diffX1X3]
  Square1/1 -> [diffX2X3]
  Square/1 -> [diffX1X2]
  Subtract2/1 -> Square2/1
  Subtract1/1 -> Square1/1
  x3/1 -> Subtract2/2, Subtract1/2
  Subtract/1 -> Square/1
  x2/1 -> Subtract/2, Subtract1/1
  x1/1 -> Subtract/1, Subtract2/1

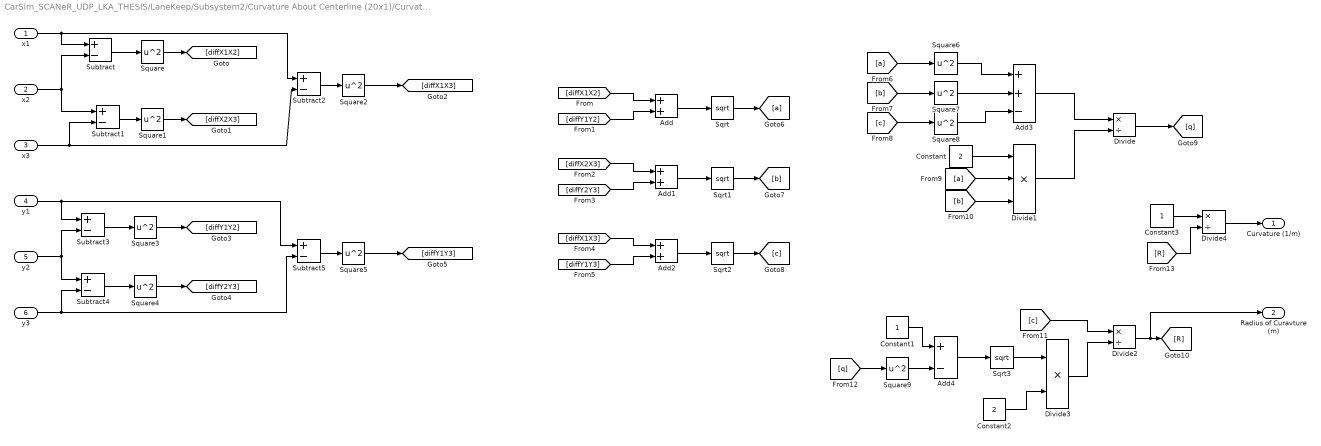
== system CarSim_SCANeR_UDP_LKA_THESIS/LaneKeep/Subsystem2/Curvature About Centerline (20x1)/Curvature from Centerline (Look Ahead)2 ==
  x1 : Inport
  x2 : Inport  Port=2
  x3 : Inport  Port=3
  y1 : Inport  Port=4
  y2 : Inport  Port=5
  y3 : Inport  Port=6
  Add : Sum
  Add1 : Sum
  Add2 : Sum
  Add3 : Sum  Inputs=++-
  Add4 : Sum  Inputs=+-
  Constant : Constant  Value=2
  Constant1 : Constant
  Constant2 : Constant  Value=2
  Constant3 : Constant
  Divide : Product  Inputs=*/
  Divide1 : Product  Inputs=***
  Divide2 : Product  Inputs=*/
  Divide3 : Product  Inputs=**
  Divide4 : Product  Inputs=*/
  Sqrt{,1..3} (4 alike) : Sqrt  SaturateOnIntegerOverflow=on
  Square{,1..9} (10 alike) : Math  Operator=square  SaturateOnIntegerOverflow=on
  Subtract{,1..5} (6 alike) : Sum  Inputs=+-
  "Curvature (1/m) " : Outport  VectorParamsAs1DForOutWhenUnconnected=on
  Radius of Curavture (m) : Outport  Port=2  VectorParamsAs1DForOutWhenUnconnected=on
  wires:
  x1/1 -> Subtract2/1, Subtract/1
  x2/1 -> Subtract1/1, Subtract/2
  Subtract/1 -> Square/1
  x3/1 -> Subtract1/2, Subtract2/2
  Subtract1/1 -> Square1/1
  Subtract2/1 -> Square2/1
  Square/1 -> [diffX1X2]
  Square1/1 -> [diffX2X3]
  Square2/1 -> [diffX1X3]
  Subtract3/1 -> Square3/1
  y1/1 -> Subtract5/1, Subtract3/1
  y2/1 -> Subtract4/1, Subtract3/2
  Subtract4/1 -> Square4/1
  y3/1 -> Subtract5/2, Subtract4/2
  Subtract5/1 -> Square5/1
  Square3/1 -> [diffY1Y2]
  Square4/1 -> [diffY2Y3]
  Square5/1 -> [diffY1Y3]
  [diffX1X2] -> Add/1
  [diffY1Y2] -> Add/2
  Add/1 -> Sqrt/1
  Sqrt/1 -> [a]
  Sqrt1/1 -> [b]
  Add1/1 -> Sqrt1/1
  [diffY2Y3] -> Add1/2
  [diffX2X3] -> Add1/1
  [diffX1X3] -> Add2/1
  [diffY1Y3] -> Add2/2
  Add2/1 -> Sqrt2/1
  Sqrt2/1 -> [c]
  [a] -> Square6/1
  Square6/1 -> Add3/1
  [b] -> Square7/1
  Square7/1 -> Add3/2
  [c] -> Square8/1
  Square8/1 -> Add3/3
  Add3/1 -> Divide/1
  Constant/1 -> Divide1/1
  [a] -> Divide1/2
  [b] -> Divide1/3
  Divide1/1 -> Divide/2
  Divide/1 -> [q]
  [c] -> Divide2/1
  [q] -> Square9/1
  Square9/1 -> Add4/2
  Constant1/1 -> Add4/1
  Add4/1 -> Sqrt3/1
  Sqrt3/1 -> Divide3/1
  Constant2/1 -> Divide3/2
  Divide3/1 -> Divide2/2
  Divide2/1 -> [R], Radius of Curavture (m)/1
  Constant3/1 -> Divide4/1
  [R] -> Divide4/2
  Divide4/1 -> "Curvature (1/m) "/1

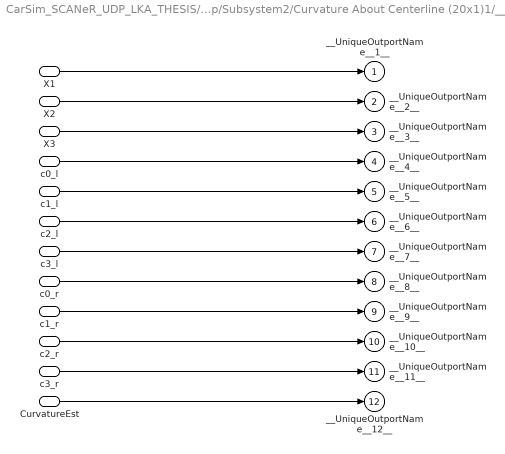
== system CarSim_SCANeR_UDP_LKA_THESIS/LaneKeep/Subsystem2/Curvature About Centerline (20x1)1/__InputSSForSFun__ ==
  X1 : Inport
  X2 : Inport  Port=2
  X3 : Inport  Port=3
  c0_l : Inport  Port=4
  c1_l : Inport  Port=5
  c2_l : Inport  Port=6
  c3_l : Inport  Port=7
  c0_r : Inport  Port=8
  c1_r : Inport  Port=9
  c2_r : Inport  Port=10
  c3_r : Inport  Port=11
  " CurvatureEst" : Inport  Port=12
  __UniqueOutportName__1__ : Outport
  __UniqueOutportName__2__ : Outport  Port=2
  __UniqueOutportName__3__ : Outport  Port=3
  __UniqueOutportName__4__ : Outport  Port=4
  __UniqueOutportName__5__ : Outport  Port=5
  __UniqueOutportName__6__ : Outport  Port=6
  __UniqueOutportName__7__ : Outport  Port=7
  __UniqueOutportName__8__ : Outport  Port=8
  __UniqueOutportName__9__ : Outport  Port=9
  __UniqueOutportName__10__ : Outport  Port=10
  __UniqueOutportName__11__ : Outport  Port=11
  __UniqueOutportName__12__ : Outport  Port=12
  wires:
  " CurvatureEst"/1 -> __UniqueOutportName__12__/1
  c3_r/1 -> __UniqueOutportName__11__/1
  c2_r/1 -> __UniqueOutportName__10__/1
  c1_r/1 -> __UniqueOutportName__9__/1
  c0_r/1 -> __UniqueOutportName__8__/1
  c3_l/1 -> __UniqueOutportName__7__/1
  c2_l/1 -> __UniqueOutportName__6__/1
  c1_l/1 -> __UniqueOutportName__5__/1
  c0_l/1 -> __UniqueOutportName__4__/1
  X3/1 -> __UniqueOutportName__3__/1
  X2/1 -> __UniqueOutportName__2__/1
  X1/1 -> __UniqueOutportName__1__/1

== system CarSim_SCANeR_UDP_LKA_THESIS/LaneKeep/Subsystem2/Curvature About Centerline (20x1)1/__OutputSSForSFun__ ==
  __UniqueInportName__1__ : Inport
  Output : Outport
  wires:
  __UniqueInportName__1__/1 -> Output/1

== matlab function CarSim_SCANeR_UDP_LKA_THESIS/LaneKeep/Subsystem2/Curvature About Centerline (20x1)/CurvatureCalculation ==
  data: x1 input; Curvature output; x2 input; x3 input; y1 input; y2 input; y3 input; RadiusOfCurvature output
function [Curvature,RadiusOfCurvature] = fcn(x1,x2,x3,y1,y2,y3)

RadiusOfCurvature = zeros(1,10);
Curvature = zeros(1,10);

for i = 1:10
    a = sqrt((x2(i)-x1(i)).^2+(y2(i)-y1(i)).^2);
    b = sqrt((x3(i)-x2(i)).^2+(y3(i)-y2(i)).^2);
    c = sqrt((x3(i)-x1(i)).^2+(y3(i)-y1(i)).^2);
    q = (a.^2+b.^2-c.^2)./(2.*a.*b);
%     q = 0.1;
    R = c/(2*sqrt(abs(1-q^2)));
    
    RadiusOfCurvature(i) = R;
    Curvature(i) = 1./R;
end

== matlab function CarSim_SCANeR_UDP_LKA_THESIS/LaneKeep/Subsystem2/Curvature About Centerline (20x1)/Y_Calculation ==
  data: c0 input; y output; c1 input; c2 input; c3 input; x input
function y = fcn(c0,c1,c2,c3,x)

y = c0+c1.*x+c2.*x.^2+c3.*x.^3;

== matlab function CarSim_SCANeR_UDP_LKA_THESIS/LaneKeep/Subsystem2/Curvature About Centerline (20x1)/Y_Calculation1 ==
  data: c0 input; y output; c1 input; c2 input; c3 input; x input
function y = fcn(c0,c1,c2,c3,x)

y = c0+c1.*x+c2.*x.^2+c3.*x.^3;

== matlab function CarSim_SCANeR_UDP_LKA_THESIS/LaneKeep/Subsystem2/Curvature About Centerline (20x1)/Y_Calculation2 ==
  data: c0 input; y output; c1 input; c2 input; c3 input; x input
function y = fcn(c0,c1,c2,c3,x)

y = c0+c1.*x+c2.*x.^2+c3.*x.^3;

== matlab function CarSim_SCANeR_UDP_LKA_THESIS/LaneKeep/Subsystem2/Curvature About Centerline (20x1)/Y_Calculation3 ==
  data: c0 input; y output; c1 input; c2 input; c3 input; x input
function y = fcn(c0,c1,c2,c3,x)

y = c0+c1.*x+c2.*x.^2+c3.*x.^3;

== matlab function CarSim_SCANeR_UDP_LKA_THESIS/LaneKeep/Subsystem2/Curvature About Centerline (20x1)/Y_Calculation4 ==
  data: c0 input; y output; c1 input; c2 input; c3 input; x input
function y = fcn(c0,c1,c2,c3,x)

y = c0+c1.*x+c2.*x.^2+c3.*x.^3;

== matlab function CarSim_SCANeR_UDP_LKA_THESIS/LaneKeep/Subsystem2/Curvature About Centerline (20x1)/Y_Calculation5 ==
  data: c0 input; y output; c1 input; c2 input; c3 input; x input
function y = fcn(c0,c1,c2,c3,x)

y = c0+c1.*x+c2.*x.^2+c3.*x.^3;

== matlab function CarSim_SCANeR_UDP_LKA_THESIS/LaneKeep/Subsystem2/Curvature About Centerline (20x1)/CurvatureCalculation2 ==
  data: x1 input; Curvature output; x2 input; x3 input; y1 input; y2 input; y3 input; RadiusOfCurvature output
function [Curvature,RadiusOfCurvature] = fcn(x1,x2,x3,y1,y2,y3)

RadiusOfCurvature = zeros(1,10);
Curvature = zeros(1,10);

for i = 1:10
    a = sqrt((x2(i)-x1(i)).^2+(y2(i)-y1(i)).^2);
    b = sqrt((x3(i)-x2(i)).^2+(y3(i)-y2(i)).^2);
    c = sqrt((x3(i)-x1(i)).^2+(y3(i)-y1(i)).^2);
    q = (a.^2+b.^2-c.^2)./(2.*a.*b);
%     q = 0.1;
    R = c/(2*sqrt(abs(1-q^2)));
    
    RadiusOfCurvature(i) = R;
    Curvature(i) = 1./R;
end

== matlab function CarSim_SCANeR_UDP_LKA_THESIS/Automate/Embedded MATLAB Function1 ==
  data: off input; regulMode output; regul input; up input; down input; speed input; inMode input; inTarget input; gearEngaged input; outMode output; outTarget output; disengage input; wantedGear output; LKA_Engage input; LKA_out output; LKA_Disengage input; LKA_out2 output; LKA_on input
function [regulMode, outMode, outTarget, wantedGear, LKA_out,LKA_out2] = fcn(off, regul, up, down, speed, inMode, inTarget,gearEngaged, disengage,LKA_Engage,LKA_Disengage,LKA_on)

ModeOff = 0;
ModeRegulOn = 1;
ModeRegulPause = 2;
minSpeed = 30;  %km/h
wantedGear = 0;

outMode = inMode;
outTarget = inTarget;

if ((regul == 1 && speed >= minSpeed) || (inMode == ModeRegulPause && (up == 1 || down == 1)))
    outMode = ModeRegulOn;
    outTarget = round(speed);
elseif inMode == ModeRegulPause && regul == 1
    outMode = ModeRegulOn;
elseif inMode == ModeRegulOn && (regul == 1 || disengage == 1)
    outMode = ModeRegulPause;
elseif inMode == ModeRegulOn && up == 1
    outTarget = inTarget + 1;
elseif inMode == ModeRegulOn && down == 1 && inTarget > minSpeed
    outTarget = inTarget - 1;
elseif off == 1
    outMode = ModeOff;
end

%Turn ACC on
if outMode == ModeRegulOn
    regulMode = 1;
    wantedGear = gearEngaged;
else
    regulMode = 0;
    wantedGear = 0;
end

%Turn LKA on

if (LKA_Engage == 1 && LKA_on == 1) || (LKA_Engage == 1 && LKA_on == 0);
    LKA_out = 1;
    LKA_out2 = 1;
elseif (LKA_Disengage == 1 && LKA_on == 1) || (LKA_Disengage == 1 && LKA_on == 0)
    LKA_out = 0;
    LKA_out2 = 0;
elseif (LKA_Engage == 0 && LKA_on == 1)
    LKA_out = 1;
    LKA_out2 = 1;
else
    LKA_out = 0;
    LKA_out2 = 0;
end
end
